simulink model "labos"  (Simulink 7.1)
settings: Solver=ode45  StartTime=0.0  StopTime=1000.0  RelTol=1e-3
settings Model: Creator=Marko Gulin  LastModifiedBy=Marko Gulin

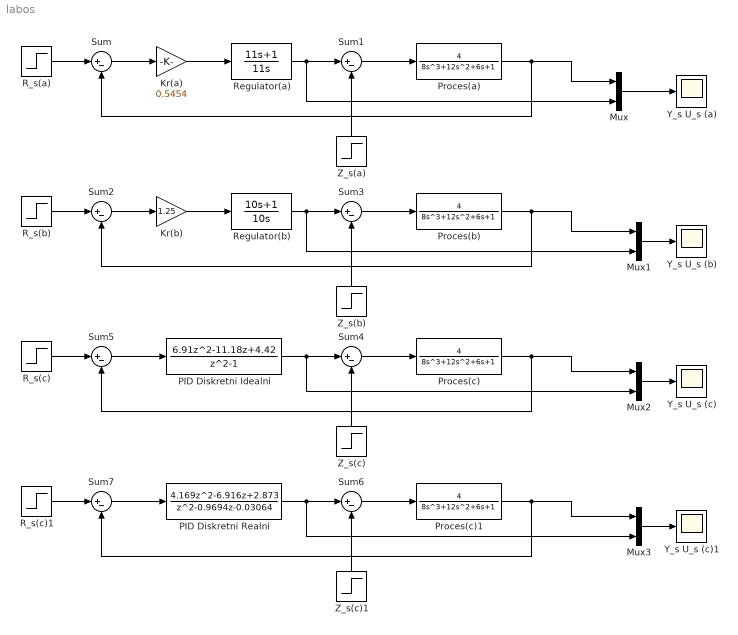
== system labos ==
  Kr(a) : Gain  Gain=0.5454  ParameterDataType=sfix(16)  ParameterScaling=2^0  OutDataType=sfix(16)  OutScaling=2^0
  Kr(b) : Gain  Gain=1.25  ParameterDataType=sfix(16)  ParameterScaling=2^0  OutDataType=sfix(16)  OutScaling=2^0
  Mux{,1..3} (4 alike) : Mux  Inputs=2
  PID Diskretni Idealni : DiscreteTransferFcn  Numerator=[6.91 -11.18 4.42]  Denominator=[1 0 -1]  SampleTime=0.37
  PID Diskretni Realni : DiscreteTransferFcn  Numerator=[4.169 -6.916 2.873]  Denominator=[1 -0.9694 -0.03064]  SampleTime=0.37
  Proces(a) : TransferFcn  Numerator=[4]  Denominator=[8 12 6 1]
  Proces(b) : TransferFcn  Numerator=[4]  Denominator=[8 12 6 1]
  Proces(c) : TransferFcn  Numerator=[4]  Denominator=[8 12 6 1]
  Proces(c)1 : TransferFcn  Numerator=[4]  Denominator=[8 12 6 1]
  R_s(a) : Step  Time=0  SampleTime=0
  R_s(b) : Step  Time=0  SampleTime=0
  R_s(c) : Step  Time=0  SampleTime=0
  R_s(c)1 : Step  Time=0  SampleTime=0
  Regulator(a) : TransferFcn  Numerator=[11 1]  Denominator=[11 0]
  Regulator(b) : TransferFcn  Numerator=[10 1]  Denominator=[10 0]
  Sum{,1..7} (8 alike) : Sum  Inputs=|+-  OutDataType=sfix(16)  OutScaling=2^0
  Y_s U_s (a) : Scope
  Y_s U_s (b) : Scope
  Y_s U_s (c) : Scope
      settings: SaveName=ScopeData2
  Y_s U_s (c)1 : Scope
      settings: SaveName=ScopeData3
  Z_s(a) : Step  Orientation=up  Time=50  SampleTime=0
  Z_s(b) : Step  Orientation=up  Time=50  SampleTime=0
  Z_s(c) : Step  Orientation=up  Time=50  SampleTime=0
  Z_s(c)1 : Step  Orientation=up  Time=50  SampleTime=0
  wires:
  Sum/1 -> Kr(a)/1
  Kr(a)/1 -> Regulator(a)/1
  Regulator(a)/1 -> Sum1/1, Mux/2
  Sum1/1 -> Proces(a)/1
  Proces(a)/1 -> Sum/2, Mux/1
  R_s(a)/1 -> Sum/1
  Z_s(a)/1 -> Sum1/2
  Sum2/1 -> Kr(b)/1
  Kr(b)/1 -> Regulator(b)/1
  Regulator(b)/1 -> Sum3/1, Mux1/2
  Sum3/1 -> Proces(b)/1
  Proces(b)/1 -> Sum2/2, Mux1/1
  R_s(b)/1 -> Sum2/1
  Z_s(b)/1 -> Sum3/2
  Mux/1 -> Y_s U_s (a)/1
  Mux1/1 -> Y_s U_s (b)/1
  PID Diskretni Idealni/1 -> Sum4/1, Mux2/2
  Sum4/1 -> Proces(c)/1
  Proces(c)/1 -> Sum5/2, Mux2/1
  Sum5/1 -> PID Diskretni Idealni/1
  R_s(c)/1 -> Sum5/1
  Z_s(c)/1 -> Sum4/2
  Mux2/1 -> Y_s U_s (c)/1
  PID Diskretni Realni/1 -> Sum6/1, Mux3/2
  Sum6/1 -> Proces(c)1/1
  Proces(c)1/1 -> Sum7/2, Mux3/1
  Sum7/1 -> PID Diskretni Realni/1
  R_s(c)1/1 -> Sum7/1
  Z_s(c)1/1 -> Sum6/2
  Mux3/1 -> Y_s U_s (c)1/1
